simulink model "SimModel"  (R2023a)
settings: Solver=VariableStepAuto  StartTime=0.0  StopTime=4  RelTol=1e-3  AbsTol=1e-3  EnableMultiTasking=on
values from neighbouring files (symbols this model uses):
  i1 = (90/18+1)^4    (= 1296)    [script.m]
  i2 = 1296    [script.m]
  i3 = (89/19+1)^4    (= 1043.95221031)    [script.m]
  i4 = 699.5    [script.m]
  Istart1 = 1.8    [script.m]
  Istart2 = 5.25    [script.m]
  Istart3 = 1.8    [script.m]
  Istart4 = 0.6    [script.m]
  isum = 3375    [script.m]
  ke = (Un-In*R)/w    (= 0.00737661998797)    [script.m]
  ke1 = (Un1-In1*R1)/w1    (= 0.0315126787322)    [script.m]
  ke2 = (Un2-In2*R2)/w2    (= 0.0370130735655)    [script.m]
  ke3 = (Un3-In3*R3)/w3    (= 0.0315126787322)    [script.m]
  ke4 = (Un4-In4*R4)/w4    (= 0.0428587508595)    [script.m]
  km = ke    (= 0.00737661998797)    [script.m]
  km1 = Mn1/In1    (= 0.0204166666667)    [script.m]
  km2 = Mn2/In2    (= 0.0204166666667)    [script.m]
  km3 = Mn3/In3    (= 0.0204166666667)    [script.m]
  km4 = Mn4/In4    (= 0.0226153846154)    [script.m]
  Kpd = 0.855    [script.m]
  R = 27.8    [script.m]
  R1 = 30    [script.m]
  R2 = 7.8    [script.m]
  R3 = 30    [script.m]
  R4 = 76.5    [script.m]
  Te = 0.1*Tm    (= 0.0063)    [script.m]
  Te1 = 0.1*Tm1    (= 0.00265782235628)    [script.m]
  Te2 = 0.1*Tm2    (= 0.00175470266366)    [script.m]
  Te3 = 0.1*Tm3    (= 0.00265782235628)    [script.m]
  Te4 = 0.1*Tm4    (= 0.00915537077571)    [script.m]
  Un = 12    [script.m]
  Un1 = 27    [script.m]
  Un2 = 27    [script.m]
  Un3 = 27    [script.m]
  Un4 = 27    [script.m]
undefined symbols (not defined in the file or in its folder): X, Y, Z
libraries: sm_lib x65, nesl_utility x21, slpidlib x11
(part 4 of 4)

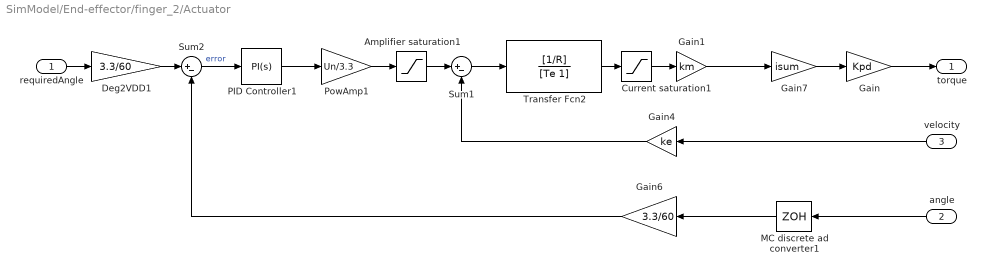
== system SimModel/End-effector/finger_2/Actuator ==
  requiredAngle : Inport
  angle : Inport  Port=2
  velocity : Inport  Port=3
  Amplifier saturation1 : Saturate  UpperLimit=12  LowerLimit=-12
  Current saturation1 : Saturate  UpperLimit=1.2  LowerLimit=-1.2
  Deg2VDD1 : Gain  Gain=3.3/60
  Gain : Gain  Gain=Kpd
  Gain1 : Gain  Gain=km
  Gain4 : Gain  Gain=ke
  Gain6 : Gain  Gain=3.3/60
  Gain7 : Gain  Gain=isum
  MC discrete ad converter1 : ZeroOrderHold  SampleTime=1e-4
  PID Controller1 : slpidlib/PID Controller  Controller=PI  Form=Parallel  TimeDomain=Continuous-time  UseExternalTs=off  SampleTime=-1  IntegratorMethod=Forward Euler  FilterMethod=Forward Euler  ControllerParametersSource=internal  P=10.8649335654251  I=0.917356238202964  UseKiTs=off  D=0  N=100  UseFilter=on  TunerSelectOption=Transfer Function Based (PID Tuner App)  InitialConditionSource=internal  InitialConditionForIntegrator=0  InitialConditionForFilter=0  DifferentiatorICPrevScaledInput=0  ExternalReset=none  TrackingMode=off  Kt=1  LimitOutput=off  SatLimitsSource=internal  UpperSaturationLimit=inf  LowerSaturationLimit=-inf  LinearizeAsGain=on  AntiWindupMode=none  Kb=1  LimitIntegrator=off  UpperIntegratorSaturationLimit=inf  LowerIntegratorSaturationLimit=-inf  POutMin=[]  POutMax=[]  IOutMin=[]  IOutMax=[]  DOutMin=[]  DOutMax=[]  NOutMin=[]  NOutMax=[]  SumOutMin=[]  SumOutMax=[]  SaturationOutMin=[]  SaturationOutMax=[]  PParamMin=[]  PParamMax=[]  IParamMin=[]  IParamMax=[]  DParamMin=[]  DParamMax=[]  NParamMin=[]  NParamMax=[]  KbParamMin=[]  KbParamMax=[]  KtParamMin=[]  KtParamMax=[]  KbOutMin=[]  KbOutMax=[]  KtOutMin=[]  KtOutMax=[]  IntegratorOutMin=[]  IntegratorOutMax=[]  FilterOutMin=[]  FilterOutMax=[]  SumI1OutMin=[]  SumI1OutMax=[]  SumI2OutMin=[]  SumI2OutMax=[]  SumI3OutMin=[]  SumI3OutMax=[]  SumI4OutMin=[]  SumI4OutMax=[]  SumDOutMin=[]  SumDOutMax=[]  DifferentiatorOutMin=[]  DifferentiatorOutMax=[]  FilterDiffOutCoefMin=[]  FilterDiffOutCoefMax=[]  ReciprocalOutMin=[]  ReciprocalOutMax=[]  SumDenOutMin=[]  SumDenOutMax=[]  SumNumOutMin=[]  SumNumOutMax=[]  DivideOutMin=[]  DivideOutMax=[]  UdiffTsProdOutMin=[]  UdiffTsProdOutMax=[]  NTsProdOutMin=[]  NTsProdOutMax=[]  UintegralTsProdOutMin=[]  UintegralTsProdOutMax=[]  UngainTsProdOutMin=[]  UngainTsProdOutMax=[]  ClampingZeroOutDataTypeStr=Inherit: Inherit via back propagation  ClampingZeroOutMin=[]  ClampingZeroOutMax=[]  FilterDenConstantOutDataTypeStr=Inherit: Inherit via back propagation  FilterDenConstantOutMin=[]  FilterDenConstantOutMax=[]  PCopyOutDataTypeStr=Inherit: Inherit via back propagation  PCopyOutMin=[]  PCopyOutMax=[]  NCopyOutDataTypeStr=Inherit: Inherit via back propagation  NCopyOutMin=[]  NCopyOutMax=[]  IntegratorContinuousStateAttributes=''  IntegratorStateMustResolveToSignalObject=off  IntegratorRTWStateStorageClass=Auto  FilterContinuousStateAttributes=''  FilterStateMustResolveToSignalObject=off  FilterRTWStateStorageClass=Auto  ParallelPVariant=InternalParameters  IdealPVariant=Disabled  IVariant=InternalParameters  DVariant=Disabled  IntegratorVariant=Continuous  SatVariant=Disabled  AWVariant=Passthrough  PCopyVariant=Disabled  TRVariant=Disabled  FdbkBlocksVariant=Forward  IdealPFdbkVariant=Disabled  SatFdbkVariant=Disabled  DerivativeFilterVariant=Disabled  NVariant=Disabled  NCopyVariant=Disabled_SignalSpec  FilterICVariant=Disabled  IntegratorICVariant=InternalICs  ExternalResetVariant=Disabled  TRSumVariant=Passthrough  SumFdbkVariant=Disabled  SumVariant=Sum_PI  TsampFilterVariant=InternalTs  TsampNgainVariant=Passthrough  TsampIntegralVariant=Disabled_SignalSpec  ExternalSaturationOutDataTypeStr=Inherit: Same as second input
  PowAmp1 : Gain  Gain=Un/3.3
  Sum1 : Sum  Inputs=|+-
  Sum2 : Sum  Inputs=|+-
  Transfer Fcn2 : TransferFcn  Numerator=[1/R]  Denominator=[Te 1]
  torque : Outport
  wires:
  Gain4/1 -> Sum1/2
  Gain1/1 -> Gain7/1
  Transfer Fcn2/1 -> Current saturation1/1
  Gain6/1 -> Sum2/2
  velocity/1 -> Gain4/1
  Deg2VDD1/1 -> Sum2/1
  Sum1/1 -> Transfer Fcn2/1
  Gain7/1 -> Gain/1
  Amplifier saturation1/1 -> Sum1/1
  PowAmp1/1 -> Amplifier saturation1/1
  requiredAngle/1 -> Deg2VDD1/1
  Current saturation1/1 -> Gain1/1
  Sum2/1 -> PID Controller1/1  "error"
  Gain/1 -> torque/1
  angle/1 -> MC discrete ad converter1/1
  MC discrete ad converter1/1 -> Gain6/1
  PID Controller1/1 -> PowAmp1/1

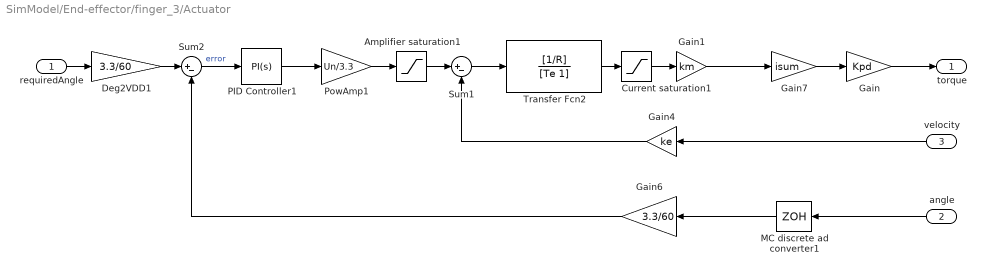
== system SimModel/End-effector/finger_3/Actuator ==
  requiredAngle : Inport
  angle : Inport  Port=2
  velocity : Inport  Port=3
  Amplifier saturation1 : Saturate  UpperLimit=12  LowerLimit=-12
  Current saturation1 : Saturate  UpperLimit=1.2  LowerLimit=-1.2
  Deg2VDD1 : Gain  Gain=3.3/60
  Gain : Gain  Gain=Kpd
  Gain1 : Gain  Gain=km
  Gain4 : Gain  Gain=ke
  Gain6 : Gain  Gain=3.3/60
  Gain7 : Gain  Gain=isum
  MC discrete ad converter1 : ZeroOrderHold  SampleTime=1e-4
  PID Controller1 : slpidlib/PID Controller  Controller=PI  Form=Parallel  TimeDomain=Continuous-time  UseExternalTs=off  SampleTime=-1  IntegratorMethod=Forward Euler  FilterMethod=Forward Euler  ControllerParametersSource=internal  P=10.8649335654251  I=0.917356238202964  UseKiTs=off  D=0  N=100  UseFilter=on  TunerSelectOption=Transfer Function Based (PID Tuner App)  InitialConditionSource=internal  InitialConditionForIntegrator=0  InitialConditionForFilter=0  DifferentiatorICPrevScaledInput=0  ExternalReset=none  TrackingMode=off  Kt=1  LimitOutput=off  SatLimitsSource=internal  UpperSaturationLimit=inf  LowerSaturationLimit=-inf  LinearizeAsGain=on  AntiWindupMode=none  Kb=1  LimitIntegrator=off  UpperIntegratorSaturationLimit=inf  LowerIntegratorSaturationLimit=-inf  POutMin=[]  POutMax=[]  IOutMin=[]  IOutMax=[]  DOutMin=[]  DOutMax=[]  NOutMin=[]  NOutMax=[]  SumOutMin=[]  SumOutMax=[]  SaturationOutMin=[]  SaturationOutMax=[]  PParamMin=[]  PParamMax=[]  IParamMin=[]  IParamMax=[]  DParamMin=[]  DParamMax=[]  NParamMin=[]  NParamMax=[]  KbParamMin=[]  KbParamMax=[]  KtParamMin=[]  KtParamMax=[]  KbOutMin=[]  KbOutMax=[]  KtOutMin=[]  KtOutMax=[]  IntegratorOutMin=[]  IntegratorOutMax=[]  FilterOutMin=[]  FilterOutMax=[]  SumI1OutMin=[]  SumI1OutMax=[]  SumI2OutMin=[]  SumI2OutMax=[]  SumI3OutMin=[]  SumI3OutMax=[]  SumI4OutMin=[]  SumI4OutMax=[]  SumDOutMin=[]  SumDOutMax=[]  DifferentiatorOutMin=[]  DifferentiatorOutMax=[]  FilterDiffOutCoefMin=[]  FilterDiffOutCoefMax=[]  ReciprocalOutMin=[]  ReciprocalOutMax=[]  SumDenOutMin=[]  SumDenOutMax=[]  SumNumOutMin=[]  SumNumOutMax=[]  DivideOutMin=[]  DivideOutMax=[]  UdiffTsProdOutMin=[]  UdiffTsProdOutMax=[]  NTsProdOutMin=[]  NTsProdOutMax=[]  UintegralTsProdOutMin=[]  UintegralTsProdOutMax=[]  UngainTsProdOutMin=[]  UngainTsProdOutMax=[]  ClampingZeroOutDataTypeStr=Inherit: Inherit via back propagation  ClampingZeroOutMin=[]  ClampingZeroOutMax=[]  FilterDenConstantOutDataTypeStr=Inherit: Inherit via back propagation  FilterDenConstantOutMin=[]  FilterDenConstantOutMax=[]  PCopyOutDataTypeStr=Inherit: Inherit via back propagation  PCopyOutMin=[]  PCopyOutMax=[]  NCopyOutDataTypeStr=Inherit: Inherit via back propagation  NCopyOutMin=[]  NCopyOutMax=[]  IntegratorContinuousStateAttributes=''  IntegratorStateMustResolveToSignalObject=off  IntegratorRTWStateStorageClass=Auto  FilterContinuousStateAttributes=''  FilterStateMustResolveToSignalObject=off  FilterRTWStateStorageClass=Auto  ParallelPVariant=InternalParameters  IdealPVariant=Disabled  IVariant=InternalParameters  DVariant=Disabled  IntegratorVariant=Continuous  SatVariant=Disabled  AWVariant=Passthrough  PCopyVariant=Disabled  TRVariant=Disabled  FdbkBlocksVariant=Forward  IdealPFdbkVariant=Disabled  SatFdbkVariant=Disabled  DerivativeFilterVariant=Disabled  NVariant=Disabled  NCopyVariant=Disabled_SignalSpec  FilterICVariant=Disabled  IntegratorICVariant=InternalICs  ExternalResetVariant=Disabled  TRSumVariant=Passthrough  SumFdbkVariant=Disabled  SumVariant=Sum_PI  TsampFilterVariant=InternalTs  TsampNgainVariant=Passthrough  TsampIntegralVariant=Disabled_SignalSpec  ExternalSaturationOutDataTypeStr=Inherit: Same as second input
  PowAmp1 : Gain  Gain=Un/3.3
  Sum1 : Sum  Inputs=|+-
  Sum2 : Sum  Inputs=|+-
  Transfer Fcn2 : TransferFcn  Numerator=[1/R]  Denominator=[Te 1]
  torque : Outport
  wires:
  Gain4/1 -> Sum1/2
  Gain1/1 -> Gain7/1
  Transfer Fcn2/1 -> Current saturation1/1
  Gain6/1 -> Sum2/2
  velocity/1 -> Gain4/1
  Deg2VDD1/1 -> Sum2/1
  Sum1/1 -> Transfer Fcn2/1
  Gain7/1 -> Gain/1
  Amplifier saturation1/1 -> Sum1/1
  PowAmp1/1 -> Amplifier saturation1/1
  requiredAngle/1 -> Deg2VDD1/1
  Current saturation1/1 -> Gain1/1
  Sum2/1 -> PID Controller1/1  "error"
  Gain/1 -> torque/1
  angle/1 -> MC discrete ad converter1/1
  MC discrete ad converter1/1 -> Gain6/1
  PID Controller1/1 -> PowAmp1/1

== matlab function SimModel/inverse kinematic ==
  data: X input; IK output; Y input; Z input; P_deg input
function IK = fcn(X,Y,Z,P_deg)

    KCI = 1; %Первоначально
    %Переведем градусы в радианы
    P = P_deg*pi/180;
    
    %Зададим матрицы поворота e
    e0 = [1 0 0; 0 1 0; 0 0 1];
    e1 = [0 0 1; 1 0 0; 0 1 0];
    e2 = [1 0 0; 0 1 0; 0 0 1];
    e3 = [1 0 0; 0 1 0; 0 0 1];
    e4 = [0 1 0; 0 0 1; 1 0 0];

    l0 = [0; 0; 0.208]; %Вектор, соединяющий 0 и 1 СК
    l1 = [0; 0.056; 0]; %Вектор, соединяющий 0 и 1 СК
    l2 = [0; 0.325; 0]; %Вектор, соединяющий 1 и 2 СК
    l3 = [0; 0.325; 0]; %Вектор, соединяющий 2 и 3 СК
    l4 = [0.013; 0.3065; 0.191]; %Вектор, соединяющий 3 и 4 СК

    
    %Рассматримаем угол поворота q1
    dx_g = 0.013; %Смещение СК4 относительно СК3 по оси X
    dy_g = 0.0095; %Смещение СК4 относительно СК3 по оси Y
    dz_g = 0.191; %Смещение СК4 относительно СК3 по оси Z
    lxy = sqrt(dx_g^2+dy_g^2); %Норма вектора смещения СК4 относительно СК3 в плоскости XY
    ldir = sqrt(X^2+Y^2-dx_g^2) - dy_g; %Норма траектории движения СК4 к заданной точке в плоскости XY
    lwan = sqrt(X^2+Y^2); %Норма вектора соединяющего СК0 и СК4 в плоскости XY
    alp = atan2(dy_g,dx_g); %Углы составляющие угол q1
    bet = atan2(Y,X);
    hama = acos((lwan^2+lxy^2-ldir^2)/(2*lwan*lxy));

    if ldir < 0
        hama = -hama;
    end

    q1 = alp + bet + hama; %Угол q1

    %Матрицы поворота одной СК относительно другой
    tau_table0 = e0; 
    tau01 = tauz(q1)*e1;
    tau_table1 = tau_table0*tau01;
    tau_1table = transpose(tau_table1);

    t4table_1 = tau_1table*[X;Y;Z]; %Вектор позиции СК4 относительно СК стола в СК1
    t41_1 = t4table_1 - l1-[0;l0(3,1);0]; %Вектор позиции СК4 относительно СК1 в СК1
    
    alp1 = atan2(dy_g,dz_g); %Угол к вертикали вектора, соединяющего СК3 и СК4
    l4xy = sqrt(dy_g^2+dz_g^2); %Норма проекции вектора, соединяющего СК3 и СК4, в плоскости XY СК1
    t31_1 = t41_1 + [l4xy*sin(P+alp1); -l4xy*cos(P+alp1); -dx_g]; %Вектор позиции СК3 относительно СК1 в СК1

    %Проведем расчет треугольника, получающийся из 2 и 3 звена
    teta = atan2(t31_1(2,1),t31_1(1,1))-pi/2;
    l23xy = sqrt(t31_1(2,1)^2+t31_1(1,1)^2);
    B = acos((l2(2,1)^2+l3(2,1)^2-l23xy^2)/(2*l2(2,1)*l3(2,1)));
    %A = acos((l2(2,1)^2-l3(2,1)^2+l23xy^2)/(2*l23xy*l2(2,1)));
    A = (pi-B)/2;
    C = A; %#ok<NASGU> 
   
    %Вычисляем обобщенные координаты
    if KCI == 1
        q2 = teta - A;
        q3 = pi - B;
        q4 = P - q2 - q3;
    else 
        q2 = teta + A;
        q3 = B - pi;
        q4 = P - q2 - q3;
    end
    
    q1_deg = q1*180/pi;
    q2_deg = q2*180/pi;
    q3_deg = q3*180/pi;
    q4_deg = q4*180/pi;

    %Приводим координаты в диапазон от -180 до 180
    if q1_deg > 180
        q1_deg = q1_deg - 360;
    end
    if q1_deg < -180
        q1_deg = 360 + q1_deg;
    end

    if q2_deg > 180
        q2_deg = q2_deg - 360;
    end
    if q2_deg < -180
        q2_deg = 360 + q2_deg;
    end

    if q3_deg > 180
        q3_deg = q3_deg - 360;
    end
    if q3_deg < -180
        q3_deg = 360 + q3_deg;
    end

    if q4_deg > 180
        q4_deg = q4_deg - 360;
    end
    if q4_deg < -180
        q4_deg = 360 + q4_deg;
    end


    if or(or(abs(q1_deg)>180, abs(q2_deg)>90), or(abs(q3_deg)>100, abs(q4_deg)>105)) %Пробуем при KCI = -1

        q2 = teta + A;
        q3 = B - pi;
        q4 = P - q2 - q3;

        q1_deg = q1*180/pi;
        q2_deg = q2*180/pi;
        q3_deg = q3*180/pi;
        q4_deg = q4*180/pi;

        if q1_deg > 180
            q1_deg = q1_deg - 360;
        end
        if q1_deg < -180
            q1_deg = 360 + q1_deg;
        end

        if q2_deg > 180
            q2_deg = q2_deg - 360;
        end
        if q2_deg < -180
            q2_deg = 360 + q2_deg;
        end

        if q3_deg > 180
            q3_deg = q3_deg - 360;
        end
        if q3_deg < -180
            q3_deg = 360 + q3_deg;
        end

        if q4_deg > 180
            q4_deg = q4_deg - 360;
        end
        if q4_deg < -180
            q4_deg = 360 + q4_deg;
        end
    end

    if or(or(abs(q1_deg)>180, abs(q2_deg)>90), or(abs(q3_deg)>100, abs(q4_deg)>105))
        q1_deg = 0;
        q2_deg = 0;
        q3_deg = 0;
        q4_deg = 0;
    end
    
    if or(or(abs(X)>0.2,Y>0),Z>0.5) %Если искомая точка вне безопасной области
        q1_deg = 0;
        q2_deg = 0;
        q3_deg = 0;
        q4_deg = 0;
    end

    if and(Z<=0.185,X^2+Y^2<=0.158^2) %Проверка на соударение с основанием
        q1_deg = 0;
        q2_deg = 0;
        q3_deg = 0;
        q4_deg = 0;
    end
    
    %Переведем градусы в радианы
    q1 = q1_deg*pi/180;
    q2 = q2_deg*pi/180;
    q3 = q3_deg*pi/180;
    q4 = q4_deg*pi/180;

    %Матрицы поворота текущей СК относительно предыдущей
    tau_table0 = e0;
    tau01 = tauz(q1)*e1;
    tau12 = tauz(q2)*e2;
    tau23 = tauz(q3)*e3;
    tau34 = tauz(q4)*e4;

    %Матрицы поворота текущей СК относистельно базовой СК стола
    tau_table1 = tau_table0*tau01;
    tau_table2 = tau_table1*tau12;
    tau_table3 = tau_table2*tau23;
    tau_table4 = tau_table3*tau34;

    t2 = tau_table0*l0 + tau_table1*l1 + tau_table2*l2;
    t3 = tau_table0*l0 + tau_table1*l1 + tau_table2*l2 + tau_table3*l3;

    if or(or(or(t3(3,1)>0.7,abs(t3(1,1))>0.2),t2(3,1)>0.7),abs(t2(1,1))>0.2) %Проверка на выход шарниров из безопасной области
        q1_deg = 0;
        q2_deg = 0;
        q3_deg = 0;
        q4_deg = 0;
    end
    %Выведем полученные значения
    q_deg = [q1_deg;q2_deg;q3_deg;q4_deg]; %#ok<> 

    %q1 = q1_deg*pi/180;
    %q2 = q2_deg*pi/180;
    %q3 = q3_deg*pi/180;
    %q4 = q4_deg*pi/180;
    
    %Для того, чтобы матрица Якоби была обратимой
    %if q3 == 0 
    %    q3 = KCI/10^5;
    %end

    %Матрицы поворота текущей СК относительно предыдущей
    %tau_table0 = e0;
    %tau01 = tauz(q1)*e1;
    %tau12 = tauz(q2)*e2;
    %tau23 = tauz(q3)*e3;
    %tau34 = tauz(q4)*e4;

    %Матрицы поворота текущей СК относистельно базовой СК стола
    %tau_table1 = tau_table0*tau01;
    %tau_table2 = tau_table1*tau12;
    %tau_table3 = tau_table2*tau23;
    %tau_table4 = tau_table3*tau34;

    %Найдем линейные скорости схвата
    %Элементы матрицы Якоби для линейных скоростей
    %D41 = lambda(tau_table1*e1'*[0; 0; 1])*(tau_table1*l1+tau_table2*l2+tau_table3*l3+tau_table4*l4); 
    %D42 = lambda(tau_table2*e2'*[0; 0; 1])*(tau_table2*l2+tau_table3*l3+tau_table4*l4);
    %D43 = lambda(tau_table3*e3'*[0; 0; 1])*(tau_table3*l3+tau_table4*l4);
    %D44 = lambda(tau_table4*e4'*[0; 0; 1])*(tau_table4*l4);
    %Якобиан для скоростей
    %J = [D41(1,1) D42(1,1) D43(1,1) D44(1,1); D41(2,1) D42(2,1) D43(2,1) D44(2,1); D41(3,1) D42(3,1) D43(3,1) D44(3,1); 0 1 1 1];
    %pq = inv(J)*[LGS(1,1); LGS(2,1); LGS(3,1); pP]; %#ok<MINV> 
    
    %Округлим, так как присутствует вычислительная ошибка и как следствие -
    %незначащие цифры
    %pq = round(pq*10)/10;

    %Выведем значение обобщенных скоростей
    %pq_degps = round(pq*1800/pi)/10; %#ok<NASGU> 

    IK = q_deg;

function res = tauz(q)
    res = [cos(q) -sin(q) 0; sin(q) cos(q) 0; 0 0 1];
    
%function res = lambda(a)
%    res = [0 -a(3,1) a(2,1); a(3,1) 0 -a(1,1); a(2,1) a(1,1) 0];
